simulink model "prac_p2"  (R2024a)
settings: Solver=VariableStepAuto  StartTime=0.0  StopTime=1000  RelTol=1e-3
libraries: simulink x1
settings Model: Creator=heman  LastModifiedBy=heman

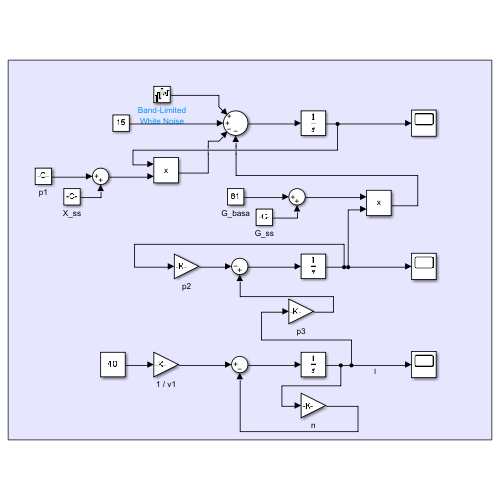
[thumbnail: Simulink's stored preview of the top-level diagram]
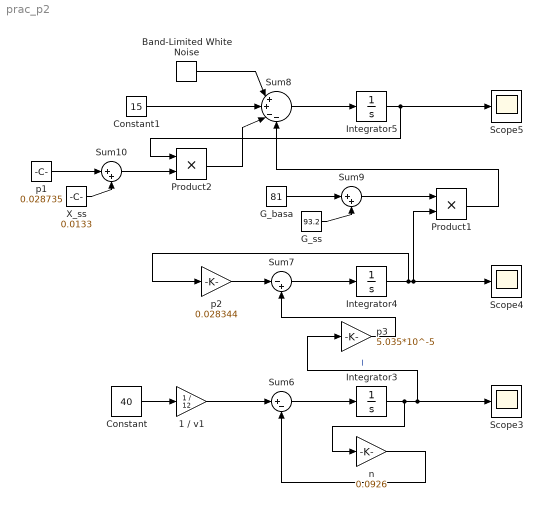
== system prac_p2 ==
  1 / v1 : Gain  Gain=1 / 12
  Band-Limited White Noise : simulink/Sources/Band-Limited White Noise  Cov=[0.1]  Ts=0.1  seed=[23341]
  Constant : Constant  Value=40
  Constant1 : Constant  Value=15
  G_basa : Constant  Value=81
  G_ss : Constant  Value=93.2
  Integrator3 : Integrator
  Integrator4 : Integrator
  Integrator5 : Integrator
  Product1 : Product
  Product2 : Product
  Scope3 : Scope
  Scope4 : Scope
  Scope5 : Scope
  Sum10 : Sum  Inputs=|++
  Sum6 : Sum  Inputs=|+-
  Sum7 : Sum  Inputs=|-+
  Sum8 : Sum  Inputs=|++--
  Sum9 : Sum  Inputs=|++
  X_ss : Constant  Value=0.0133
  n : Gain  Gain=0.0926
  p1 : Constant  Value=0.028735
  p2 : Gain  Gain=0.028344
  p3 : Gain  Gain=5.035*10^-5
  wires:
  p3/1 -> Sum7/2
  p2/1 -> Sum7/1
  n/1 -> Sum6/2
  Sum9/1 -> Product1/1
  Sum6/1 -> Integrator3/1
  Integrator3/1 -> n/1, p3/1, Scope3/1  "I"
  Sum7/1 -> Integrator4/1
  X_ss/1 -> Sum10/2
  p1/1 -> Sum10/1
  G_ss/1 -> Sum9/2
  Constant1/1 -> Sum8/2
  G_basa/1 -> Sum9/1
  Sum8/1 -> Integrator5/1
  Integrator5/1 -> Product2/1, Scope5/1
  Constant/1 -> 1 / v1/1
  Sum10/1 -> Product2/2
  Product2/1 -> Sum8/3
  Integrator4/1 -> p2/1, Product1/2, Scope4/1
  1 / v1/1 -> Sum6/1
  Product1/1 -> Sum8/4
  Band-Limited White Noise/1 -> Sum8/1
